simulink library "Library"  (R2017b)
settings: Solver=ode45  StartTime=0.0  StopTime=10.0  RelTol=1e-3  EnableMultiTasking=on
values from neighbouring files (symbols this model uses):
  PLL_tau = 1/500    (= 0.002)    [dataaustralian14gen.m]
  visat = inf    [dataaustralian14gen.m]
undefined symbols (not defined in the file or in its folder): j, Ki, Kp
libraries: powerlib x15, powerlib_meascontrol x2
settings Model: Creator=Philipp  LastModifiedBy=dominic
settings DataIOCC: LimitDataPoints=on
settings OptimizationCC: LifeSpan=inf
settings DebuggingCC: AllowSymbolicDim=off  SFUnexpectedBacktrackingDiag=warning  SFNoUnconditionalDefaultTransitionDiag=warning  SFExecutionAtInitializationDiag=none
settings CodeAppCC: StateflowObjectComments=on
settings GRTTargetCC: TargetLangStandard=C89/C90 (ANSI)  GeneratePreprocessorConditionals=Disable all
settings ConfigComp: CovMetricSettings=dw  CovHtmlReporting=on  CovSaveCumulativeToWorkspaceVar=on  CovSaveSingleToWorkspaceVar=on  CovExternalEMLEnable=off

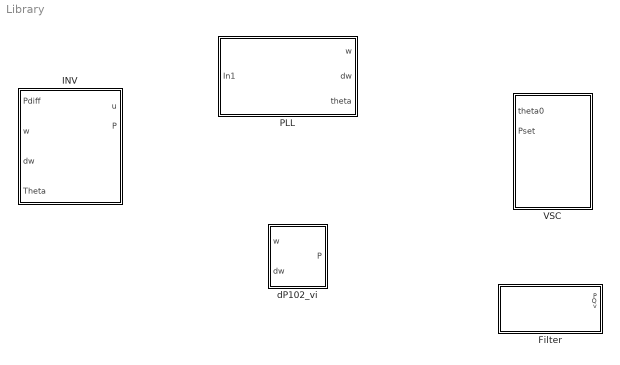
== system Library ==
  Filter : Subsystem  mask{r=0, l=0, c=0}
  INV : Subsystem  mask{fn=50, Ub=20e3, Pref=0, ang=0, K2=1e2, K1=1}
      mask prompts: fn "Frequency (Hz)"; Ub "Base Voltage (V)"; Pref "Power Ref [W]"; ang "initial angle (deg)"; K2 "D/M"; K1 "1/M"
  PLL : Subsystem  mask(Phase Locked Loop){Kp=Kp, Ki=Ki, tau=PLL_tau, theta0=0, omega0=0}
      mask prompts: Kp "Proportional Control Parameter (Kp)"; Ki "Integral Control Parameter (Ki)"; tau "filter time constant"; theta0 "initial angle (deg)"; omega0 "initial frequency (rad/s)"
  VSC : Subsystem
  dP102_vi : Subsystem  mask{d=0, m=0}
      mask prompts: d "Damping"; m "Inertia"

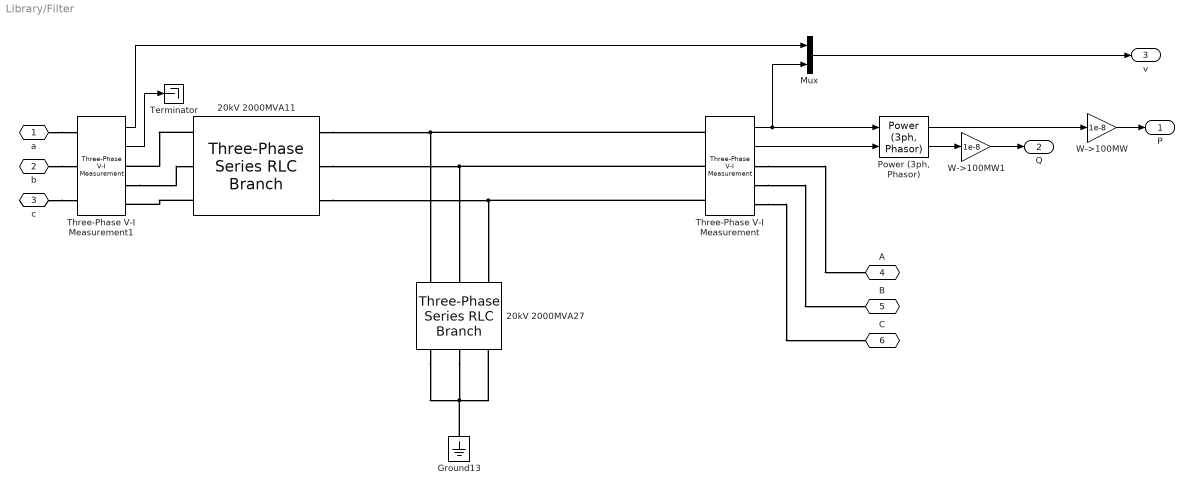
== system Library/Filter ==
  20kV 2000MVA11 : powerlib/Elements/Three-Phase Series RLC Branch  LConnTagsString=A|B|C  RConnTagsString=A|B|C  BranchType=RL  Resistance=r  Inductance=l  Capacitance=[]  Measurements=None
  20kV 2000MVA27 : powerlib/Elements/Three-Phase Series RLC Branch  LConnTagsString=A|B|C  RConnTagsString=A|B|C  BranchType=C  Resistance=20^2/2000  Inductance=20^2/2000  Capacitance=c  Measurements=None
  Ground13 : powerlib/Elements/Ground  LConnTagsString=a
  Mux : Mux  Inputs=2
  "Power (3ph, Phasor)" : powerlib_meascontrol/Measurements/Power (3ph, Phasor)
      settings: SourceProductName=Simscape Power Systems  SourceProductBaseCode=PS
  Terminator : Terminator
  Three-Phase V-I Measurement : powerlib/Measurements/Three-Phase V-I Measurement  VoltageMeasurement=phase-to-ground  SetLabelV=off  LabelV=Vabc  Vpu=off  VpuLL=off  CurrentMeasurement=yes  SetLabelI=off  LabelI=Iabc  Ipu=off  Pbase=100e6  Vbase=500e3  OutputType=Complex  PhasorSimulation=on  PSBequivalent=0
  Three-Phase V-I Measurement1 : powerlib/Measurements/Three-Phase V-I Measurement  VoltageMeasurement=phase-to-ground  SetLabelV=off  LabelV=Vabc  Vpu=off  VpuLL=off  CurrentMeasurement=yes  SetLabelI=off  LabelI=Iabc  Ipu=off  Pbase=100e6  Vbase=500e3  OutputType=Complex  PhasorSimulation=on  PSBequivalent=0
  W->100MW : Gain  Gain=1e-8
  W->100MW1 : Gain  Gain=1e-8
  a : PMIOPort  Port=1  Side=Left
  b : PMIOPort  Port=2  Side=Left
  c : PMIOPort  Port=3  Side=Left
  A : PMIOPort  Tag=PMCPort  Port=4  Side=Right
  B : PMIOPort  Tag=PMCPort  Port=5  Side=Right
  C : PMIOPort  Tag=PMCPort  Port=6  Side=Right
  P : Outport
  Q : Outport  Port=2
  v : Outport  Port=3
  wires:
  Three-Phase V-I Measurement/2 -> "Power (3ph, Phasor)"/2
  "Power (3ph, Phasor)"/1 -> W->100MW/1
  "Power (3ph, Phasor)"/2 -> W->100MW1/1
  Three-Phase V-I Measurement/1 -> Mux/2, "Power (3ph, Phasor)"/1
  W->100MW1/1 -> Q/1
  W->100MW/1 -> P/1
  Three-Phase V-I Measurement1/2 -> Terminator/1
  Three-Phase V-I Measurement1/1 -> Mux/1
  Mux/1 -> v/1
  connections:
  20kV 2000MVA11/RConn2 -- Three-Phase V-I Measurement/LConn2 -- 20kV 2000MVA27/RConn2
  20kV 2000MVA11/RConn3 -- Three-Phase V-I Measurement/LConn3 -- 20kV 2000MVA27/RConn3
  20kV 2000MVA11/RConn1 -- Three-Phase V-I Measurement/LConn1 -- 20kV 2000MVA27/RConn1
  20kV 2000MVA27/LConn2 -- 20kV 2000MVA27/LConn3 -- Ground13/LConn1 -- 20kV 2000MVA27/LConn1
  Three-Phase V-I Measurement/RConn1 -- A/RConn1
  Three-Phase V-I Measurement/RConn2 -- B/RConn1
  Three-Phase V-I Measurement/RConn3 -- C/RConn1
  a/RConn1 -- Three-Phase V-I Measurement1/LConn1
  b/RConn1 -- Three-Phase V-I Measurement1/LConn2
  c/RConn1 -- Three-Phase V-I Measurement1/LConn3
  20kV 2000MVA11/LConn1 -- Three-Phase V-I Measurement1/RConn1
  Three-Phase V-I Measurement1/RConn2 -- 20kV 2000MVA11/LConn2
  20kV 2000MVA11/LConn3 -- Three-Phase V-I Measurement1/RConn3

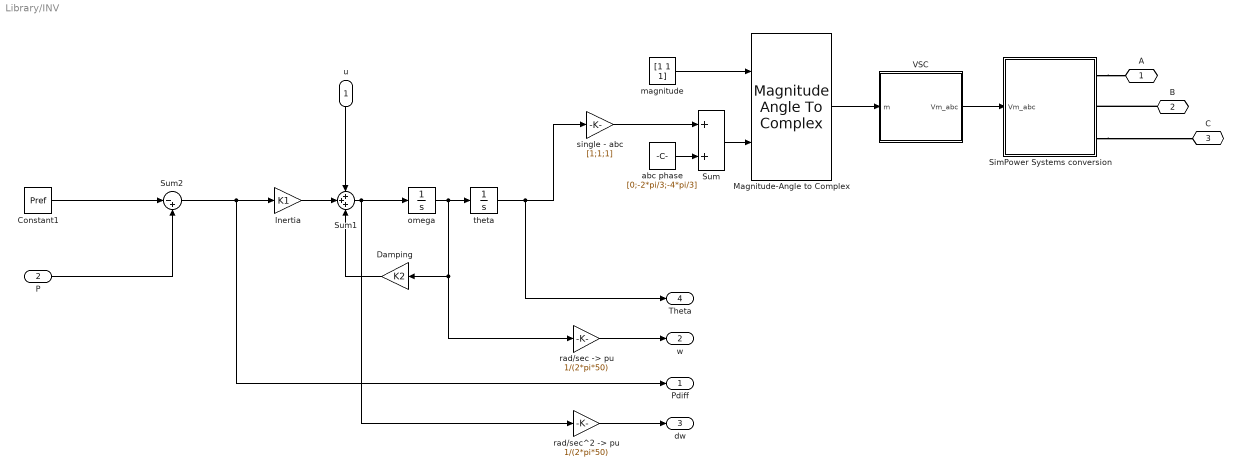
== system Library/INV ==
  u : Inport
  P : Inport  Port=2
  Constant1 : Constant  Value=Pref
  Damping : Gain  Gain=K2
  Inertia : Gain  Gain=K1
  Magnitude-Angle to Complex : MagnitudeAngleToComplex
  SimPower Systems conversion : Subsystem
      mask Display:
      | plot(0,0,100,100, [10,10,90,90,10,10,40,10,10,40,10,10,90,90,90,60,90],[90,10,10,90,90,50,50,70,30,50,50,10,10,70,70,50,30])
      | disp('SPS')
  Sum : Sum
  Sum1 : Sum  Inputs=+++
  Sum2 : Sum  Inputs=|-+
  VSC : Subsystem  mask(Hacheur){}
  abc phase : Constant  Value=[0;-2*pi/3;-4*pi/3]
  magnitude : Constant  Value=[1 1 1]
  omega : Integrator
  "rad/sec -> pu" : Gain  Gain=1/(2*pi*50)
  "rad/sec^2 -> pu" : Gain  Gain=1/(2*pi*50)
  single - abc : Gain  Gain=[1;1;1]
  theta : Integrator  InitialCondition=ang/180*pi
  A : PMIOPort  Tag=PMCPort  Port=1  Side=Left
  B : PMIOPort  Tag=PMCPort  Port=2  Side=Left
  C : PMIOPort  Tag=PMCPort  Port=3  Side=Left
  Pdiff : Outport
  w : Outport  Port=2
  dw : Outport  Port=3
  Theta : Outport  Port=4
  wires:
  VSC/1(Vm_abc) -> SimPower Systems conversion/1(Vm_abc)
  Magnitude-Angle to Complex/1 -> VSC/1(m)
  magnitude/1 -> Magnitude-Angle to Complex/1
  omega/1 -> Damping/1, "rad/sec -> pu"/1, theta/1
  abc phase/1 -> Sum/2
  single - abc/1 -> Sum/1
  Sum/1 -> Magnitude-Angle to Complex/2
  Sum1/1 -> omega/1, "rad/sec^2 -> pu"/1
  theta/1 -> Theta/1, single - abc/1
  Constant1/1 -> Sum2/1
  Inertia/1 -> Sum1/2
  Damping/1 -> Sum1/3
  u/1 -> Sum1/1
  Sum2/1 -> Pdiff/1, Inertia/1
  "rad/sec -> pu"/1 -> w/1
  "rad/sec^2 -> pu"/1 -> dw/1
  P/1 -> Sum2/2
  connections:
  SimPower Systems conversion/RConn1 -- A/RConn1
  B/RConn1 -- SimPower Systems conversion/RConn2
  SimPower Systems conversion/RConn3 -- C/RConn1

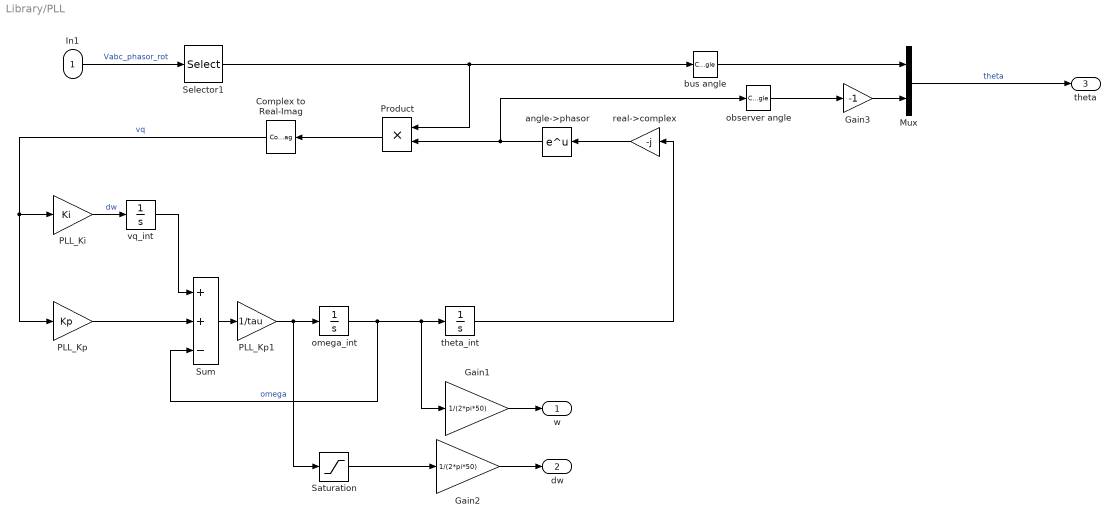
== system Library/PLL ==
  In1 : Inport
  Complex to Real-Imag : ComplexToRealImag  Output=Imag
  Gain1 : Gain  Gain=1/(2*pi*50)
  Gain2 : Gain  Gain=1/(2*pi*50)
  Gain3 : Gain  Gain=-1
  Mux : Mux  Inputs=2
  PLL_Ki : Gain  Gain=Ki
  PLL_Kp : Gain  Gain=Kp
  PLL_Kp1 : Gain  Gain=1/tau
  Product : Product
  Saturation : Saturate  UpperLimit=6*2*pi  LowerLimit=-6*2*pi
  Selector1 : Selector  InputPortWidth=3  IndexOptions=Index vector (dialog)  Indices=1  OutputSizes=1
  Sum : Sum  Inputs=++-
  angle->phasor : Math  SaturateOnIntegerOverflow=on
  bus angle : ComplexToMagnitudeAngle  Output=Angle
  observer angle : ComplexToMagnitudeAngle  Output=Angle
  omega_int : Integrator  InitialCondition=omega0
  real->complex : Gain  Gain=-j
  theta_int : Integrator  InitialCondition=theta0/180*pi
  vq_int : Integrator
  w : Outport
  dw : Outport  Port=2
  theta : Outport  Port=3
  wires:
  real->complex/1 -> angle->phasor/1
  omega_int/1 -> Sum/3, Gain1/1, theta_int/1  "omega"
  theta_int/1 -> real->complex/1
  angle->phasor/1 -> observer angle/1, Product/2
  observer angle/1 -> Gain3/1
  bus angle/1 -> Mux/1
  In1/1 -> Selector1/1  "Vabc_phasor_rot"
  Product/1 -> Complex to Real-Imag/1
  Selector1/1 -> bus angle/1, Product/1
  Complex to Real-Imag/1 -> PLL_Kp/1, PLL_Ki/1  "vq"
  Gain3/1 -> Mux/2
  Gain1/1 -> w/1
  Gain2/1 -> dw/1
  Mux/1 -> theta/1  "theta"
  Sum/1 -> PLL_Kp1/1
  Saturation/1 -> Gain2/1
  PLL_Kp/1 -> Sum/2
  PLL_Ki/1 -> vq_int/1  "dw"
  vq_int/1 -> Sum/1
  PLL_Kp1/1 -> Saturation/1, omega_int/1

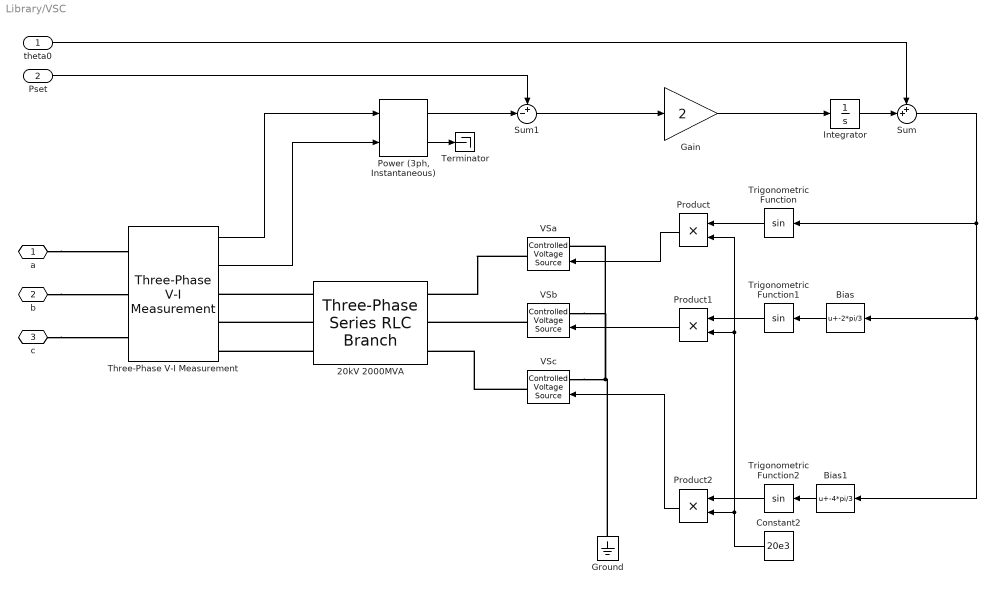
== system Library/VSC ==
  theta0 : Inport
  Pset : Inport  Port=2
  20kV 2000MVA : powerlib/Elements/Three-Phase Series RLC Branch  LConnTagsString=A|B|C  RConnTagsString=A|B|C  BranchType=RL  Resistance=20^2/2000/10  Inductance=20^2/2000/377  Capacitance=[]  Measurements=None
  Bias : Bias  Bias=-2*pi/3
  Bias1 : Bias  Bias=-4*pi/3
  Constant2 : Constant  Value=20e3
  Gain : Gain  Gain=2
  Ground : powerlib/Elements/Ground  LConnTagsString=a
  Integrator : Integrator
  "Power (3ph, Instantaneous)" : powerlib_meascontrol/Measurements/Power (3ph, Instantaneous)
      settings: SourceProductName=Simscape Power Systems
  Product : Product
  Product1 : Product
  Product2 : Product
  Sum : Sum  Inputs=++|
  Sum1 : Sum  Inputs=+-|
  Terminator : Terminator
  Three-Phase V-I Measurement : powerlib/Measurements/Three-Phase V-I Measurement  VoltageMeasurement=phase-to-ground  SetLabelV=off  LabelV=Vabc  Vpu=off  VpuLL=off  CurrentMeasurement=yes  SetLabelI=off  LabelI=Iabc  Ipu=off  Pbase=100e6  Vbase=500e3  OutputType=Complex  PhasorSimulation=off  PSBequivalent=0
  Trigonometric Function : Trigonometry
  Trigonometric Function1 : Trigonometry
  Trigonometric Function2 : Trigonometry
  VSa : powerlib/Electrical Sources/Controlled Voltage Source  Initialize=on  Source_Type=AC  Amplitude=0  Phase=0  Frequency=0  Measurements=None
  VSb : powerlib/Electrical Sources/Controlled Voltage Source  Initialize=on  Source_Type=AC  Amplitude=0  Phase=0  Frequency=0  Measurements=None
  VSc : powerlib/Electrical Sources/Controlled Voltage Source  Initialize=on  Source_Type=AC  Amplitude=0  Phase=0  Frequency=0  Measurements=None
  a : PMIOPort  Port=1  Side=Left
  b : PMIOPort  Port=2  Side=Left
  c : PMIOPort  Port=3  Side=Left
  wires:
  Bias/1 -> Trigonometric Function1/1
  Product1/1 -> VSb/1
  Trigonometric Function1/1 -> Product1/1
  Three-Phase V-I Measurement/2 -> "Power (3ph, Instantaneous)"/2
  "Power (3ph, Instantaneous)"/2 -> Terminator/1
  Product2/1 -> VSc/1
  Three-Phase V-I Measurement/1 -> "Power (3ph, Instantaneous)"/1
  Trigonometric Function2/1 -> Product2/1
  Constant2/1 -> Product/2, Product1/2, Product2/2
  Gain/1 -> Integrator/1
  Trigonometric Function/1 -> Product/1
  Product/1 -> VSa/1
  Bias1/1 -> Trigonometric Function2/1
  Sum/1 -> Trigonometric Function/1, Bias1/1, Bias/1
  Integrator/1 -> Sum/2
  theta0/1 -> Sum/1
  "Power (3ph, Instantaneous)"/1 -> Sum1/2
  Sum1/1 -> Gain/1
  Pset/1 -> Sum1/1
  connections:
  20kV 2000MVA/LConn1 -- Three-Phase V-I Measurement/RConn1
  VSb/RConn1 -- 20kV 2000MVA/RConn2
  VSa/RConn1 -- 20kV 2000MVA/RConn1
  20kV 2000MVA/LConn2 -- Three-Phase V-I Measurement/RConn2
  VSc/RConn1 -- 20kV 2000MVA/RConn3
  20kV 2000MVA/LConn3 -- Three-Phase V-I Measurement/RConn3
  VSc/LConn1 -- Ground/LConn1 -- VSb/LConn1 -- VSa/LConn1
  b/RConn1 -- Three-Phase V-I Measurement/LConn2
  a/RConn1 -- Three-Phase V-I Measurement/LConn1
  c/RConn1 -- Three-Phase V-I Measurement/LConn3

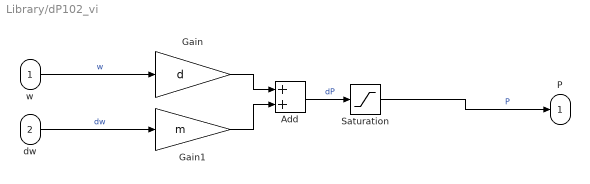
== system Library/dP102_vi ==
  w : Inport
  dw : Inport  Port=2
  Add : Sum
  Gain : Gain  Gain=d
  Gain1 : Gain  Gain=m
  Saturation : Saturate  UpperLimit=visat  LowerLimit=-visat  ZeroCross=off
  P : Outport
  wires:
  Gain1/1 -> Add/2
  Gain/1 -> Add/1
  dw/1 -> Gain1/1  "dw"
  w/1 -> Gain/1  "w"
  Add/1 -> Saturation/1  "dP"
  Saturation/1 -> P/1  "P"

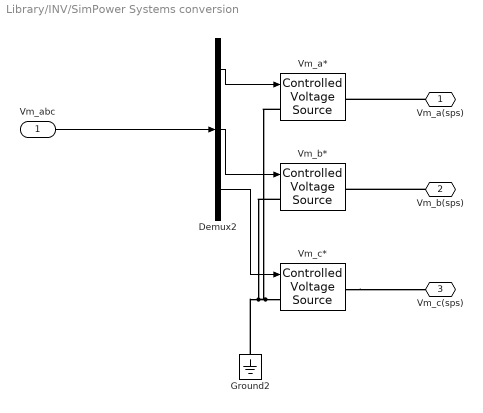
== system Library/INV/SimPower Systems conversion ==
  Vm_abc : Inport
  Demux2 : Demux  Outputs=3
  Ground2 : powerlib/Elements/Ground  LConnTagsString=a
  Vm_a* : powerlib/Electrical Sources/Controlled Voltage Source  Initialize=on  Source_Type=AC  Amplitude=Ub*sqrt(2/3)  Phase=ang  Frequency=fn  Measurements=None
  Vm_b* : powerlib/Electrical Sources/Controlled Voltage Source  Initialize=on  Source_Type=AC  Amplitude=Ub*sqrt(2/3)  Phase=ang-120  Frequency=fn  Measurements=None
  Vm_c* : powerlib/Electrical Sources/Controlled Voltage Source  Initialize=on  Source_Type=AC  Amplitude=Ub*sqrt(2/3)  Phase=ang-240  Frequency=fn  Measurements=None
  Vm_a(sps) : PMIOPort  Port=1  Side=Right
  Vm_b(sps) : PMIOPort  Port=2  Side=Right
  Vm_c(sps) : PMIOPort  Port=3  Side=Right
  wires:
  Demux2/3 -> Vm_c*/1
  Demux2/1 -> Vm_a*/1
  Vm_abc/1 -> Demux2/1
  Demux2/2 -> Vm_b*/1
  connections:
  Vm_c*/LConn1 -- Vm_b*/LConn1 -- Vm_a*/LConn1 -- Ground2/LConn1
  Vm_c*/RConn1 -- Vm_c(sps)/RConn1
  Vm_b(sps)/RConn1 -- Vm_b*/RConn1
  Vm_a(sps)/RConn1 -- Vm_a*/RConn1

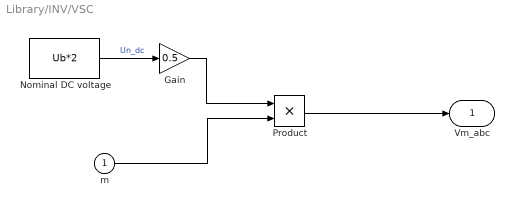
== system Library/INV/VSC ==
  m : Inport
  Gain : Gain  Gain=0.5
  Nominal DC voltage : Constant  Value=Ub*2
  Product : Product  RndMeth=Zero
  Vm_abc : Outport  InitialOutput=0
  wires:
  Nominal DC voltage/1 -> Gain/1  "Un_dc"
  m/1 -> Product/2
  Product/1 -> Vm_abc/1
  Gain/1 -> Product/1
